simulink model "BFsimple"  (R2015a)
settings: Solver=ode45  StartTime=0.0  StopTime=10.0  RelTol=1e-6
values from neighbouring files (symbols this model uses):
  h = lsim(m.ee,u,t)    [Modeles.m]    (also in Parametres.m = 0.06)
undefined symbols (not defined in the file or in its folder): m
settings Model: Creator=David  LastModifiedBy=David
settings DataIOCC: LimitDataPoints=off

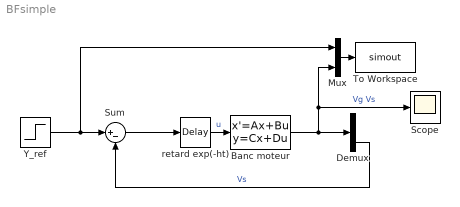
== system BFsimple ==
  Banc moteur : StateSpace  A=m.ee.a  B=m.ee.b  C=m.ee.c  D=m.ee.d  X0=0
  Demux : Demux  Outputs=2
  Mux : Mux  Inputs=2
  Scope : Scope
  Sum : Sum  Inputs=|+-
  To Workspace : ToWorkspace  VariableName=simout  SaveFormat=Structure With Time  SampleTime=-1
  Y_ref : Step  Time=0  SampleTime=0
  retard exp(-ht) : TransportDelay  DelayTime=h
  wires:
  Y_ref/1 -> Mux/1, Sum/1
  retard exp(-ht)/1 -> Banc moteur/1  "u"
  Banc moteur/1 -> Mux/2, Scope/1, Demux/1  "Vg Vs"
  Demux/2 -> Sum/2  "Vs"
  Sum/1 -> retard exp(-ht)/1
  Mux/1 -> To Workspace/1
